simulink model "zhengliu"  (R2019b)
settings: Solver=ode23tb  StartTime=0.0  StopTime=0.05  RelTol=1e-3  EnableMultiTasking=on
undefined symbols (not defined in the file): D11, Delta
libraries: powerlib x18, powerlib_extras x4
settings Model: Creator=Administrator  LastModifiedBy=bhisma
settings DataIOCC: LimitDataPoints=on  SaveFormat=Array  SignalLoggingSaveFormat=ModelDataLogs  ReturnWorkspaceOutputs=off  SignalLoggingName=sigsOut
settings OptimizationCC: InitFltsAndDblsToZero=on  LifeSpan=inf
settings DebuggingCC: SaveWithParameterizedLinksMsg=none  UnderspecifiedInitializationDetection=Classic  MergeDetectMultiDrivingBlocksExec=none  SignalResolutionControl=TryResolveAllWithWarning  MultiTaskDSMMsg=warning  MultiTaskCondExecSysMsg=none  FcnCallInpInsideContextMsg=warning  AllowSymbolicDim=off  SFUnexpectedBacktrackingDiag=warning  SFNoUnconditionalDefaultTransitionDiag=warning  SFExecutionAtInitializationDiag=none  ArithmeticOperatorsInVariantConditions=warning
settings HardwareCC: ProdBitPerPointer=32  ProdBitPerSizeT=32  ProdBitPerPtrDiffT=32  ProdLargestAtomicFloat=None  ProdIntDivRoundTo=Undefined  ProdEndianess=Unspecified  ProdWordSize=32  ProdHWDeviceType=32-bit Generic  TargetUnknown=on
settings ModelReferenceCC: PropagateSignalLabelsOutOfModel=off
settings SFSimCC: SimUseLocalCustomCode=off  CustomCodeUndefinedFunction=UseInterfaceOnly
settings RTWCC: RTWUseLocalCustomCode=off
settings CodeAppCC: StateflowObjectComments=on
settings GRTTargetCC: TargetFcnLib=ansi_tfl_tmw.mat  TargetLangStandard=C89/C90 (ANSI)  CombineOutputUpdateFcns=off  GRTInterface=on
settings ConfigComp: CovMetricSettings=dw  CovHtmlReporting=on  CovSaveCumulativeToWorkspaceVar=on  CovSaveSingleToWorkspaceVar=on  CovExternalEMLEnable=off
settings SimscapeCC: SimscapeNormalizeSystem=off

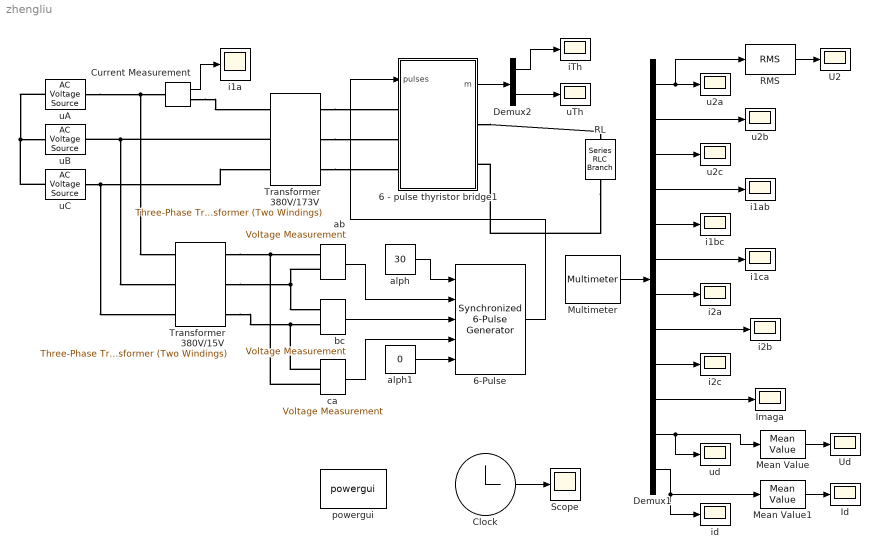
== system zhengliu ==
  " RL" : powerlib/Elements/Series RLC Branch  LConnTagsString=__new0  RConnTagsString=__new0  BranchType=RL  Resistance=0.5  Inductance=0.01  SetiL0=off  InitialCurrent=0  Capacitance=[]  Setx0=off  InitialVoltage=0  Measurements=Branch voltage and current
      settings: SourceProductName=Simscape Electrical
  6 - pulse thyristor bridge1 : Subsystem  AncestorBlock=|  mask(Six-pulse thyristor bridge){Ron=0.01, Lon=10e-6, Rs=2000, Cs=50e-9}
      | powerlib_extras/Three-Phase
      | Library/6 - pulse
      |  thyristor bridge
      mask prompts: Ron "Thyristor on-state resitance (Ohms) :"; Lon "Thyristor on-state inductance (H) :"; Rs "Snubber resistance (Ohms) :"; Cs "Snubber capacitance (F) :"
      mask help:
      | This block implements a six-pulses thyristor bridge rectifier with RC snubbers. Set the snubber resistance to Inf to remove all the thyristors snubbers. This block uses six Simplified Thyristors from the powerlib/Power Electronics library.
      | Input four (labeled 'pulses') of the block is a Simulink vector of length six that  controls the thyristors gates. Use the 'Look Under Mask' in the Edit menu  to see how the control vector operates the six thyrsistors.
      mask init:
      | power_initmask();
      settings: OpenFcn=power_openblockproxy()
      mask Display: plot(0,0,100,100,[50,50,35,50,65,50],[30,40,40,60,40,40],[35,65],[60,60],[50,50],[60,70],[45,40],[60,65],[35,40],[65,65])
  6-Pulse : powerlib_extras/Control  Blocks/Synchronized 6-Pulse Generator  freq=50  pwidth=10  Double_Pulse=on
      settings: SourceProductName=Simscape Electrical  SourceProductBaseCode=PS
  Clock : Clock
  Current Measurement : powerlib/Measurements/Current Measurement  PhasorSimulation=off  OutputType=Complex  PSBequivalent=0
      settings: SourceProductName=Simscape Electrical
  Demux1 : Demux  Outputs=12
  Demux2 : Demux  Outputs=2
  Id : Scope
  Imaga : Scope
  Mean Value : powerlib_extras/Measurements/Mean Value  Period=1/60
      settings: SourceProductName=Simscape Electrical  SourceProductBaseCode=PS
  Mean Value1 : powerlib_extras/Measurements/Mean Value  Period=1/60
      settings: SourceProductName=Simscape Electrical  SourceProductBaseCode=PS
  Multimeter : powerlib/Measurements/Multimeter  PhasorSimulation=off  OutputType=Magnitude  sel=[5 6 7 9 10 11 12 13 14 18 1 8]  L=23  Gain=[1 1 1 1 1 1 1 1 1 1 1 1]  yselected="{'Uan_w2: Transformer 380V//173V','Ubn_w2: Transformer 380V//173V','Ucn_w2: Transformer 380V//173V','Iab_w1: Transformer 380V//173V','Ibc_w1: Transformer 380V//173V','Ica_w1: Transformer 380V//173V','Ian_w2: Transformer 380V//173V','Ibn_w2: Transformer 380V//173V','Icn_w2: Transformer 380V//173V','Imag_A: Transformer 380V//173V','Ub:  RL','Ib:  RL'};"  PSBOutputType=1  PSBequivalent=0  AxesSetting=[0,0.1,-100,100]  Display=0  SavedBlockNames=-11
      settings: SourceProductName=Simscape Electrical
  RMS : powerlib_extras/Measurements/RMS  f1=60
      settings: SourceProductName=Simscape Electrical  SourceProductBaseCode=PS
  Scope : Scope
  Transformer 380V/15V : powerlib/Elements/Three-Phase Transformer (Two Windings)  Winding1Connection=Delta (D11)  Winding2Connection=Y  CoreType=Three single-phase transformers  SetSaturation=off  Hysteresis=off  DataFile='hysteresis'  SetInitialFlux=off  Measurements=None  UNITS=pu  NominalPower=[ 250e6 , 60 ]  Winding1=[ 380 , 0.002 , 0.08 ]  Winding2=[ 15 , 0.002 , 0.08 ]  Rm=500  Lm=500  L0=0.5  Saturation=[ 0,0 ; 0.0024,1.2 ; 1.0,1.52 ]  InitialFluxes=[ 0.8 , -0.8 , 0.7 ]  BreakLoop=off  DiscreteSolver=Trapezoidal iterative  DataType=off  TransfoNumber=0
      settings: SourceProductName=Simscape Electrical
  Transformer 380V/173V : powerlib/Elements/Three-Phase Transformer (Two Windings)  Winding1Connection=Delta (D11)  Winding2Connection=Y  CoreType=Three single-phase transformers  SetSaturation=off  Hysteresis=off  DataFile='hysteresis'  SetInitialFlux=off  Measurements=All measurements (V I Fluxes)  UNITS=pu  NominalPower=[ 250e6 , 50 ]  Winding1=[ 380 , 0.02 , 0 ]  Winding2=[ 173 , 0.02 , 0]  Rm=inf  Lm=150000  L0=0.5  Saturation=[ 0,0 ; 0.0024,1.2 ; 1.0,1.52 ]  InitialFluxes=[ 0.8 , -0.8 , 0.7 ]  BreakLoop=off  DiscreteSolver=Trapezoidal iterative  DataType=off  TransfoNumber=0
      settings: SourceProductName=Simscape Electrical
  U2 : Scope
  Ud : Scope
  ab : powerlib/Measurements/Voltage Measurement  PhasorSimulation=off  OutputType=Magnitude  PSBequivalent=0
      settings: SourceProductName=Simscape Electrical
  alph : Constant  Value=30
  alph1 : Constant  Value=0
  bc : powerlib/Measurements/Voltage Measurement  PhasorSimulation=off  OutputType=Magnitude  PSBequivalent=0
      settings: SourceProductName=Simscape Electrical
  ca : powerlib/Measurements/Voltage Measurement  PhasorSimulation=off  OutputType=Magnitude  PSBequivalent=0
      settings: SourceProductName=Simscape Electrical
  i1a : Scope
  i1ab : Scope
  i1bc : Scope
  i1ca : Scope
  i2a : Scope
  i2b : Scope
  i2c : Scope
  iTh : Scope
  "id " : Scope
  powergui : powerlib/powergui  Priority=1  SimulationMode=Continuous  SampleTime=50e-6  frequency=60  Iterations=50  frequencyindice=50  Pbase=100e6  ErrMax=1e-4  UnitsV=kV  UnitsW=MW  buscounter=0  FunctionMessages=off  echomessages=off  EnableUseOfTLC=off  CurrentSourceSwitches=off  DisableSnubberDevices=off  DisableRonSwitches=off  DisableVfSwitches=off  DisplayEquations=off  AutomaticDiscreteSolvers=off  SolverType=Tustin/Backward Euler (TBE)  Interpol=off  ExternalGateDelay=off  methode=off  Ts=10  x0status=blocks  SPID=off  SwTol=0  HookPort=off  NonlinearTolerance=1e-4  nMaxIteration=100  ContinueOnMaxIteration=off  RestoreLinks=warning  ResistiveCurrentMeasurement=off  Frange=[0:2:500]  Ylog=off  Xlog=on  ShowGrid=off  save=off  variable=ZData  structure=0  ZoomFFT=off  StartTime=0.0  cycles=1  DisplayStyle=1  fundamental=60  FreqAxis=off  MaxFrequency=1000  frequencyindicesteady=1  RmsSteady=1  display=off
      settings: SourceProductName=Simscape Electrical
  u2a : Scope
  u2b : Scope
  u2c : Scope
  uA : powerlib/Electrical Sources/AC Voltage Source  Amplitude=220*sqrt(2)  Phase=0  Frequency=50  SampleTime=0  Measurements=None  BusType=swing  Pref=10e3  Qref=0  Qmin=-inf  Qmax=+inf
      settings: SourceProductName=Simscape Electrical
  uB : powerlib/Electrical Sources/AC Voltage Source  Amplitude=220*sqrt(2)  Phase=-120  Frequency=50  SampleTime=0  Measurements=None  BusType=swing  Pref=10e3  Qref=0  Qmin=-inf  Qmax=+inf
      settings: SourceProductName=Simscape Electrical
  uC : powerlib/Electrical Sources/AC Voltage Source  Amplitude=220*sqrt(2)  Phase=-240  Frequency=50  SampleTime=0  Measurements=None  BusType=swing  Pref=10e3  Qref=0  Qmin=-inf  Qmax=+inf
      settings: SourceProductName=Simscape Electrical
  uTh : Scope
  ud : Scope
  wires:
  Multimeter/1 -> Demux1/1
  ab/1 -> 6-Pulse/2
  bc/1 -> 6-Pulse/3
  ca/1 -> 6-Pulse/4
  alph/1 -> 6-Pulse/1
  alph1/1 -> 6-Pulse/5
  6-Pulse/1 -> 6 - pulse thyristor bridge1/1(pulses)
  Demux1/1 -> u2a/1, RMS/1
  Demux1/2 -> u2b/1
  Demux1/3 -> u2c/1
  Demux1/4 -> i1ab/1
  Demux1/5 -> i1bc/1
  Demux1/6 -> i1ca/1
  Demux1/7 -> i2a/1
  Demux1/10 -> Imaga/1
  Demux1/8 -> i2b/1
  Demux1/9 -> i2c/1
  Mean Value/1 -> Ud/1
  Demux1/11 -> ud/1, Mean Value/1
  Demux1/12 -> "id "/1, Mean Value1/1
  RMS/1 -> U2/1
  Mean Value1/1 -> Id/1
  6 - pulse thyristor bridge1/1(m) -> Demux2/1
  Demux2/1 -> iTh/1
  Demux2/2 -> uTh/1
  Current Measurement/1 -> i1a/1
  Clock/1 -> Scope/1
  connections:
  uA/RConn1 -- Transformer 380V/15V/LConn1 -- Current Measurement/LConn1
  Transformer 380V/173V/LConn2 -- uB/RConn1 -- Transformer 380V/15V/LConn2
  uC/RConn1 -- Transformer 380V/15V/LConn3 -- Transformer 380V/173V/LConn3
  ca/LConn2 -- ab/LConn1 -- Transformer 380V/15V/RConn1
  ab/LConn2 -- bc/LConn1 -- Transformer 380V/15V/RConn2
  ca/LConn1 -- bc/LConn2 -- Transformer 380V/15V/RConn3
  uC/LConn1 -- uA/LConn1 -- uB/LConn1
  6 - pulse thyristor bridge1/RConn1 -- " RL"/LConn1
  Transformer 380V/173V/RConn1 -- 6 - pulse thyristor bridge1/LConn1
  Transformer 380V/173V/RConn2 -- 6 - pulse thyristor bridge1/LConn2
  Transformer 380V/173V/RConn3 -- 6 - pulse thyristor bridge1/LConn3
  Current Measurement/RConn1 -- Transformer 380V/173V/LConn1
  " RL"/RConn1 -- 6 - pulse thyristor bridge1/RConn2

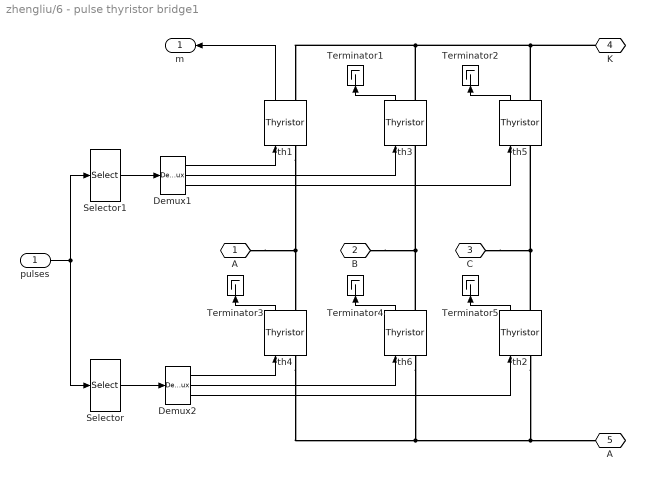
== system zhengliu/6 - pulse thyristor bridge1 ==
  pulses : Inport
  Demux1 : Demux  Outputs=3
  Demux2 : Demux  Outputs=3
  Selector : Selector  InputPortWidth=6  IndexOptions=Index vector (dialog)  Indices=[ 4 6 2]  OutputSizes=1
  Selector1 : Selector  InputPortWidth=6  IndexOptions=Index vector (dialog)  Indices=[ 1 3 5]  OutputSizes=1
  Terminator{1..5} (5 alike) : Terminator
  th{1..6} (6 alike) : powerlib/Power Electronics/Thyristor  Ron=Ron  Lon=Lon  Vf=0  IC=0  Rs=Rs  Cs=Cs  Measurements=on
      settings: SourceProductName=Simscape Electrical
  A : PMIOPort  Side=Left
  B : PMIOPort  Port=2  Side=Left
  C : PMIOPort  Port=3  Side=Left
  "K " : PMIOPort  Port=4  Side=Right
  "A " : PMIOPort  Port=5  Side=Right
  m : Outport
  wires:
  Selector/1 -> Demux2/1
  Selector1/1 -> Demux1/1
  pulses/1 -> Selector1/1, Selector/1
  th3/1 -> Terminator1/1
  th2/1 -> Terminator5/1
  th6/1 -> Terminator4/1
  th4/1 -> Terminator3/1
  Demux1/3 -> th5/1
  Demux1/2 -> th3/1
  Demux1/1 -> th1/1
  th1/1 -> m/1
  Demux2/1 -> th4/1
  Demux2/2 -> th6/1
  Demux2/3 -> th2/1
  th5/1 -> Terminator2/1
  connections:
  th4/LConn1 -- th6/LConn1 -- "A "/RConn1 -- th2/LConn1
  th1/LConn1 -- A/RConn1 -- th4/RConn1
  th6/RConn1 -- B/RConn1 -- th3/LConn1
  th2/RConn1 -- C/RConn1 -- th5/LConn1
  "K "/RConn1 -- th5/RConn1 -- th3/RConn1 -- th1/RConn1
